simulink model "tau2"  (R2023a)
settings: Solver=VariableStepAuto  StartTime=0.0  StopTime=0.05  RelTol=1e-3
libraries: simulink x2, spsRMSLib x1
settings Model: Creator=User  LastModifiedBy=Администратор

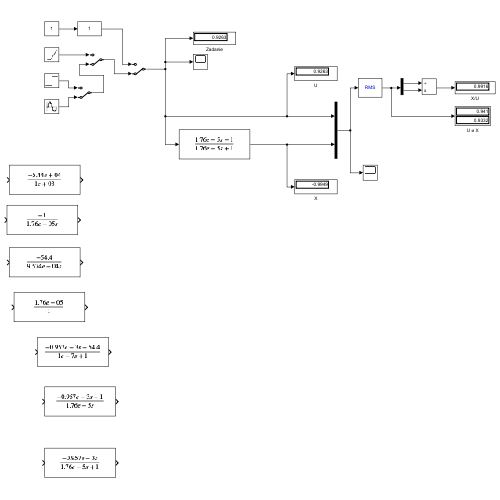
[thumbnail: Simulink's stored preview of the top-level diagram]
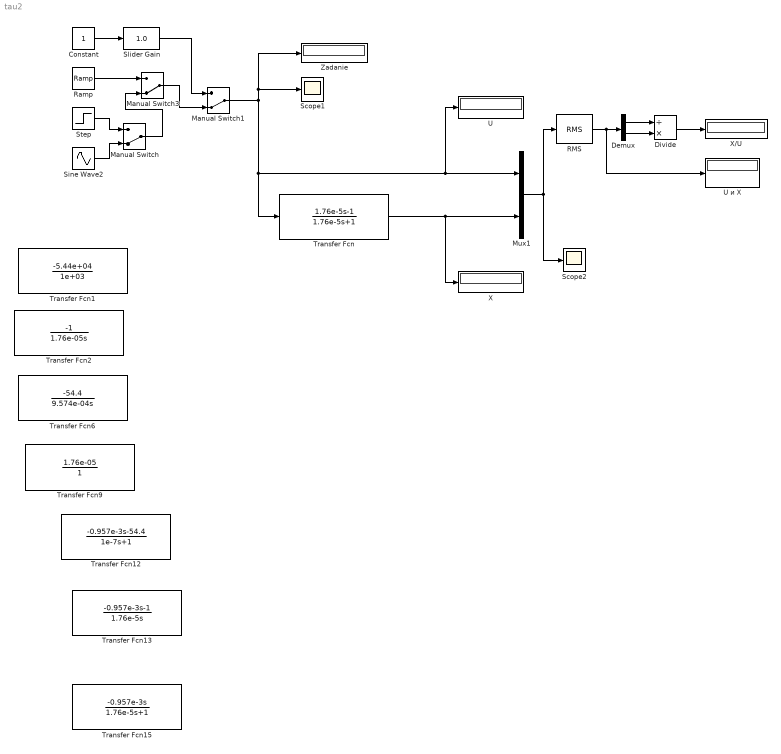
== system tau2 ==
  Constant : Constant
  Demux : Demux  Outputs=2
  Divide : Product  Inputs=/*  RndMeth=Zero  SaturateOnIntegerOverflow=on
  Manual Switch : ManualSwitch  CurrentSetting=0
  Manual Switch1 : ManualSwitch  CurrentSetting=0
  Manual Switch3 : ManualSwitch  CurrentSetting=0
  Mux1 : Mux  Inputs=2
  RMS : spsRMSLib/RMS  TrueRMS=on  Freq=1000  RMSInit=0  Ts=10^(-6)
  Ramp : simulink/Sources/Ramp  slope=1  start=0  InitialOutput=0
  Scope1 : Scope
  Scope2 : Scope
  Sine Wave2 : Sin  Frequency=166.23*2*pi  SampleTime=0.0001
  Slider Gain : simulink/Math Operations/Slider Gain  gain=1.0  low=0  high=1
  Step : Step  Time=0  SampleTime=0
  Transfer Fcn : TransferFcn  Numerator=[1.76e-5 -1]  Denominator=[1.76e-5 1]
  Transfer Fcn1 : TransferFcn  Numerator=[0 -5.44e+04]  Denominator=[0 1e+03]
  Transfer Fcn12 : TransferFcn  Numerator=[-0.957e-3 -54.4]  Denominator=[1e-7 1]
  Transfer Fcn13 : TransferFcn  Numerator=[-0.957e-3 -1]  Denominator=[1.76e-5 0]
  Transfer Fcn15 : TransferFcn  Numerator=[-0.957e-3 0]  Denominator=[1.76e-5 1]
  Transfer Fcn2 : TransferFcn  Numerator=[0 -1]  Denominator=[1.76e-05 0]
  Transfer Fcn6 : TransferFcn  Numerator=[0 -54.4]  Denominator=[9.574e-04 0]
  Transfer Fcn9 : TransferFcn  Numerator=[1.76e-05]  Denominator=[1]
  U : Display
  U и X : Display
  X : Display
  X/U : Display
  Zadanie : Display
  wires:
  Constant/1 -> Slider Gain/1
  Slider Gain/1 -> Manual Switch1/1
  Ramp/1 -> Manual Switch3/1
  Manual Switch3/1 -> Manual Switch1/2
  Step/1 -> Manual Switch/1
  Sine Wave2/1 -> Manual Switch/2
  Manual Switch/1 -> Manual Switch3/2
  Demux/2 -> Divide/2
  Demux/1 -> Divide/1
  Divide/1 -> X/U/1
  RMS/1 -> U и X/1, Demux/1
  Manual Switch1/1 -> Scope1/1, Zadanie/1, U/1, Mux1/1, Transfer Fcn/1
  Mux1/1 -> Scope2/1, RMS/1
  Transfer Fcn/1 -> Mux1/2, X/1
